simulink model "LFC_ANFIS"  (R2018a)
settings: Solver=VariableStepAuto  StartTime=0.0  StopTime=30  RelTol=1e-3
libraries: fuzblock x1
settings Model: Creator=User  LastModifiedBy=User

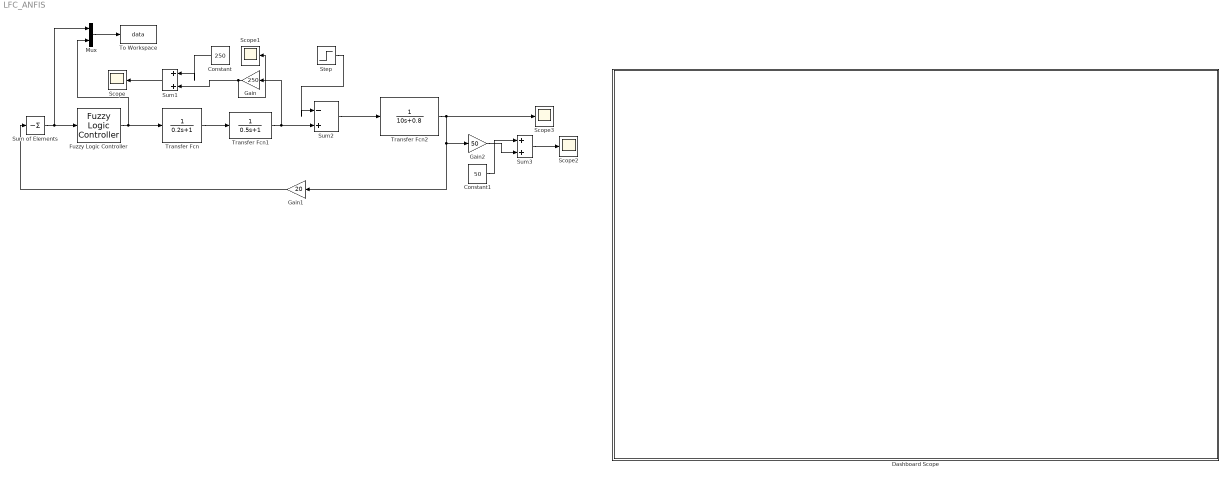
== system LFC_ANFIS ==
  Constant : Constant  Value=250
  Constant1 : Constant  Value=50
  Dashboard Scope : Subsystem  DialogController=hmiCreateDDGDialog  IsWebBlock=on  mask(MWDashboardBlock){webBlockId=11eb89da-a25d-49b4-a882-6f8da54efad0, webBlockType=sdiscope, ShowInitialText=on, HMISrcModelName=LFC_ANFIS}
      mask prompts: webBlockId "WebBlock Id"; webBlockType "WebBlock Type"; HMISrcModelName "Source Model"
      mask help: SimulinkHMI:dialogs:HMIScopeDialogDesc
      mask Help: helpview([docroot '/mapfiles/simulink.map'], 'hmi_scope')
      mask Display:
      | if strcmp(get_param(bdroot(gcb),'BlockDiagramType'), 'library')
      |     image([(matlabroot) '/toolbox/simulink/hmi/icons/DashboardScope.png']);
      | end
  Fuzzy Logic Controller : fuzblock/Fuzzy Logic  Controller  FIS='LFCneuro.fis'  OutputSampleNumber=101  DataType=double  FuzzifiedInputs=off  RuleFiringStrengths=off  RuleOutputs=off  AggregatedOutputs=off  SimulateUsing=Interpreted execution  OutOfRangeInputValueMessage=warning  NoRuleFiredMessage=warning  EmptyOutputFuzzySetMessage=warning
  Gain : Gain  Gain=250
  Gain1 : Gain  Gain=20
  Gain2 : Gain  Gain=50
  Mux : Mux  Inputs=2
  Scope{,1..3} (4 alike) : Scope
  Step : Step  SampleTime=0
  Sum of Elements : Sum  Inputs=-
  Sum1 : Sum  Inputs=|++
  Sum2 : Sum  Inputs=|-+
  Sum3 : Sum  Inputs=|++
  To Workspace : ToWorkspace  VariableName=data  SampleTime=-1
  Transfer Fcn : TransferFcn  Denominator=[0.2 1]
  Transfer Fcn1 : TransferFcn  Denominator=[0.5 1]
  Transfer Fcn2 : TransferFcn  Denominator=[10 0.8]
  wires:
  Transfer Fcn/1 -> Transfer Fcn1/1
  Transfer Fcn1/1 -> Gain/1, Sum2/2
  Sum2/1 -> Transfer Fcn2/1
  Step/1 -> Sum2/1
  Gain/1 -> Scope1/1, Sum1/2
  Constant/1 -> Sum1/1
  Sum1/1 -> Scope/1
  Constant1/1 -> Sum3/1
  Transfer Fcn2/1 -> Scope3/1, Gain1/1, Gain2/1
  Sum3/1 -> Scope2/1
  Gain2/1 -> Sum3/2
  Gain1/1 -> Sum of Elements/1
  Sum of Elements/1 -> Fuzzy Logic Controller/1, Mux/1
  Mux/1 -> To Workspace/1
  Fuzzy Logic Controller/1 -> Mux/2, Transfer Fcn/1

== system LFC_ANFIS/Dashboard Scope ==
